simulink model "backupmodelforfutureuse24jan_2012b"  (R2012b)
settings: Solver=ode45  StartTime=0.0  StopTime=10.0  RelTol=1e-3
settings Model: Creator=Vicon  LastModifiedBy=Vicon

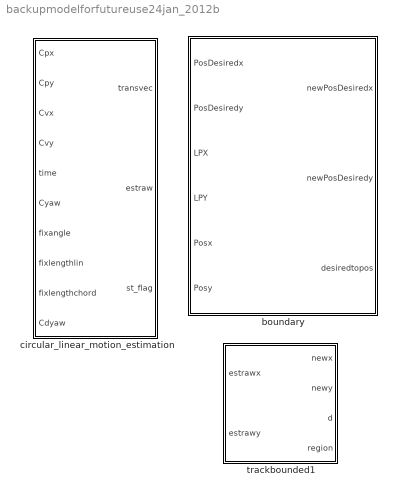
== system backupmodelforfutureuse24jan_2012b ==
  boundary : MATLAB Function  TreatAsAtomicUnit=on
  circular_linear_motion_estimation : MATLAB Function  TreatAsAtomicUnit=on
  trackbounded1 : MATLAB Function  TreatAsAtomicUnit=on

== matlab function backupmodelforfutureuse24jan_2012b/circular_linear_motion_estimation ==
  data: Cpx input; Cpy input; Cvx input; Cvy input; transvec output; estraw output; st_flag output; time input; Cyaw input; fixangle input; fixlengthlin input; fixlengthchord input; Cdyaw input
function [transvec,estraw,st_flag] = fcn(Cpx,Cpy,Cvx,Cvy,time,Cyaw,fixangle,fixlengthlin,fixlengthchord,Cdyaw)
if(Cvx == 0 && Cvy == 0)
    st_flag = 1;
else 
    st_flag = 0;
end
%%%%%%%%%%%%%%%%%%%%%%circular estimation%%%%%%%%%%%%%%%%%%%%%%%%%%%%
%vxyM = sqrt((Cvx)^2 + (Cvy)^2); %resultant vector vxy
if(st_flag == 0)
    
        angleOmega = Cyaw + 0.5 * fixangle * pi / 180; %angleOmega(radian): between vx and L
        zero_chk = 1;
else
    
      angleOmega = 0;  
      zero_chk = 0;
end
if(Cdyaw ~= 0) %use dyaw to select circular or linear estimation
%r = vxyM / abs(Cdyaw);
%Chord = 2 * r * sin(fixangle * pi / 360); %%%%%chord sometime will go to
%very large value, will disable this parameter soon
transveccir = [fixlengthchord * cos(angleOmega)*zero_chk  fixlengthchord * sin(angleOmega) * zero_chk];
transveclin = [0 0];
else
%%%%%%%%%%%%%%%%%%%%%%%%linear estimation%%%%%%%%%%%%%%%%%%%%%%%%%%%%%%
transveclin = [fixlengthlin * cos(Cyaw * pi / 180)*zero_chk fixlengthlin * sin(Cyaw * pi / 180)*zero_chk];
transveccir = [0 0];
%Chord = 0;
end
if(time<2)       %%%%%%%%%%%%%%%%%avoid noise when initializing the program in first 2 seconds
    transvec = [0 0];
else
transvec = transveccir + transveclin;
end

C2dvec = [Cpx Cpy];
estraw = C2dvec + transvec;

== matlab function backupmodelforfutureuse24jan_2012b/trackbounded1 ==
  data: newx output; newy output; estrawx input; estrawy input; d output; region output
function [newx,newy,d,region]  = fcn(estrawx,estrawy)
%#codegen
%cp = [cpy,cpx,0];
cpest = [estrawy, estrawx,0];
%%database of check points
chk0x = -0.4383;
chk0y = -0.9285;
chk1x = 1.047;
chk1y = -0.9693;
chk2x = 1.396;
chk2y = 0.4535;
chk3x = 1.382;
chk3y = 1.505;
chk4x = 1.042;
chk4y = 1.925;
chk5x = 0.3708;
chk5y = 1.821;
%%chk5x = ;
%%chk....
chk0 = [chk0y,chk0x,0];
chk1 = [chk1y,chk1x,0];
chk2 = [chk2y,chk2x,0];
chk3 = [chk3y,chk3x,0];
chk4 = [chk4y,chk4x,0];
chk5 = [chk5y,chk5x,0];
%%%%%%%%%%%%%%%%%%%%%%%%%%%%%%%%%%%%%%%%%%%%%%%%%%%%%%%%%%%%%%%%%%%%%%%%%%%%%%%%%%%%%%region selector
if(estrawx>2 && estrawx<=3 && estrawy>-3 && estrawy<=-2)
    region = 0;
elseif(estrawx>2 && estrawx<=3 && estrawy>-2 && estrawy<=-1 )
    region = 1;
elseif(estrawx>2 && estrawx<=3 && estrawy>-1 && estrawy<=0 )
    region = 2;
elseif(estrawx>2 && estrawx<=3 && estrawy>0 && estrawy<=1 )
    region = 3;
elseif(estrawx>2 && estrawx<=3 && estrawy>1 && estrawy<=2)
    region = 4;
elseif(estrawx>2 && estrawx<=3 && estrawy>2 && estrawy<=3)
    region = 5;
elseif(estrawx>1 && estrawx<=2 && estrawy>-3 && estrawy<=-2)
    region = 6;
elseif(estrawx>1 && estrawx<=2 && estrawy>-2 && estrawy<=-1)
    region = 7;
elseif(estrawx>1 && estrawx<=2 && estrawy>-1 && estrawy<=0)
    region = 8;
elseif(estrawx>1 && estrawx<=2 && estrawy>0 && estrawy<=1)
    region = 9;
elseif(estrawx>1 && estrawx<=2 && estrawy>1 && estrawy<=2)
    region = 10;
elseif(estrawx>1 && estrawx<=2 && estrawy>2 && estrawy<=3)
    region = 11;
elseif(estrawx>0 && estrawx<=1 && estrawy>-3 && estrawy<=-2)
    region = 12;
elseif(estrawx>0 && estrawx<=1 && estrawy>-2 && estrawy<=-1)
    region = 13;
elseif(estrawx>0 && estrawx<=1 && estrawy>-1 && estrawy<=0)
    region = 14;
elseif(estrawx>0 && estrawx<=1 && estrawy>0 && estrawy<=1)
    region = 15;
elseif(estrawx>0 && estrawx<=1 && estrawy>1 && estrawy<=2)
    region = 16;
elseif(estrawx>0 && estrawx<=1 && estrawy>2 && estrawy<=3)
    region = 17;
elseif(estrawx>-1 && estrawx<=0 && estrawy>-3 && estrawy<=-2)
    region = 18;
elseif(estrawx>-1 && estrawx<=0 && estrawy>-2 && estrawy<=-1)
    region = 19;
elseif(estrawx>-1 && estrawx<=0 && estrawy>-1 && estrawy<=0)
    region = 20;
elseif(estrawx>-1 && estrawx<=0 && estrawy>0 && estrawy<=1)
    region = 21;
elseif(estrawx>-1 && estrawx<=0 && estrawy>1 && estrawy<=2)
    region = 22;
elseif(estrawx>-1 && estrawx<=0 && estrawy>2 && estrawy<=3)
    region = 23;
elseif(estrawx>-2 && estrawx<=-1 && estrawy>-3 && estrawy<=-2)
    region = 24;
elseif(estrawx>-2 && estrawx<=-1 && estrawy>-2 && estrawy<=-1)
    region = 25;
elseif(estrawx>-2 && estrawx<=-1 && estrawy>-1 && estrawy<=0)
    region = 26;
elseif(estrawx>-2 && estrawx<=-1 && estrawy>0 && estrawy<=1)
    region = 27;
elseif(estrawx>-2 && estrawx<=-1 && estrawy>1 && estrawy<=2)
    region = 28;
elseif(estrawx>-2 && estrawx<=-1 && estrawy>2 && estrawy<=3)
    region = 29;
elseif(estrawx>-3 && estrawx<=-2 && estrawy>-3 && estrawy<=-2)
    region = 30;
elseif(estrawx>-3 && estrawx<=-2 && estrawy>-2 && estrawy<=-1)
    region = 31;
elseif(estrawx>-3 && estrawx<=-2 && estrawy>-1 && estrawy<=0)
    region = 32;
elseif(estrawx>-3 && estrawx<=-2 && estrawy>0 && estrawy<=1)
    region = 33;
elseif(estrawx>-3 && estrawx<=-2 && estrawy>1 && estrawy<=2)
    region = 34;
elseif(estrawx>-3 && estrawx<=-2 && estrawy>2 && estrawy<=3)
    region = 35;
else
    region = -1;
end
%%%%%%%%%%%%%%%%%%%%%%%%%%%%%%%%%%%%%%%%%%%%%%%%%%%%%%%%%%%%%%%%%%%%%%%%%%%%%%%%%%%%%%%%%%%%%%%%%%
if(region == 20 || region==19||region==13||region==14||region==7||region==21||region==6||region==12||region==18||region==24||region==25||region==26||region==27)
    %%%%%%%%%%%%%%%%calculate point to line distance%%%%%%%%%%%
    a = chk1 - chk0;
    b = cpest - chk0;
    d = norm(cross(a,b)) / norm(a);
    angle = atan2((chk1x-chk0x),(chk1y-chk0y));
    samplex = chk0x;
    sampley = chk0y;
    samplefinalx = chk1x;
    samplefinaly = chk1y;
    zero = 1;
elseif(region == 2||region==1||region==0||region==8)
    a = chk2 - chk1;
    b = cpest - chk1;
    d = norm(cross(a,b)) / norm(a);
    angle = atan2((chk2x-chk1x),(chk2y-chk1y));
    zero = 1;
    samplex = chk1x;
    sampley = chk1y;
    samplefinalx = chk2x;
    samplefinaly = chk2y;
elseif(region == 3||region==9||region==15)
    a = chk3 - chk2;
    b = cpest - chk2;
    d = norm(cross(a,b)) / norm(a);
    angle = atan2((chk3x-chk2x),(chk3y-chk2y));
    zero = 1;
    samplex = chk2x;
    sampley = chk2y;
    samplefinalx = chk3x;
    samplefinaly = chk3y;
elseif(region == 5||region==5||region==10||region==11)
    a = chk4 - chk3;
    b = cpest - chk3;
    d = norm(cross(a,b)) / norm(a);
    angle = atan2((chk4x-chk3x),(chk4y-chk3y));
    zero = 1;  
    samplex = chk3x;
    sampley = chk3y;
    samplefinalx = chk4x;
    samplefinaly = chk4y;
elseif(region == 16||region==17||region==22||region==23||region==28||region==29||region==34||region==35)
    a = chk5 - chk4;
    b = cpest - chk4;
    d = norm(cross(a,b)) / norm(a);
    angle = atan2((chk5x-chk4x),(chk5y-chk4y));
    zero = 1;
     samplex = chk4x;
    sampley = chk4y;
    samplefinalx = chk5x;
    samplefinaly = chk5y;

else
    a = -1;
    b = -1;
    d = -1;
    angle = -1;%%% i know this is not correct i will add one more zero coefficient to cancel this case
    zero = 0;
    samplex = 0;
    sampley = 0;
    samplefinalx = 0;
    samplefinaly = 0;
end
%%%%%%%%%%%%%%%%%%%%%%%%%%%%%%%%%%%%%%%%%%%%%%%%%%%%%%%%%%%%%%%%%%%%%%%%%%%%%%%%%%%%%%%%%%%%%%%%%%
%%calculate project point on the check point line
if(region == -1)%%if out of boundary none of the region match
        newy = 0;
        newx = 0;
else   %%match the region

distance = sqrt((samplefinalx-estrawx)^2+(samplefinaly-estrawy)^2); 
%if(distance > 1)
    %newx = samplefinalx;
   % newy = samplefinaly;
%else
      if(d<0.75)%%test the boundary width normal case if less than 0.75 m
    newx = estrawx;
    newy = estrawy;
      else%% out of boundary
        if(angle == 0 ||angle == 180)
            newx  = samplex;
            newy = estrawy;
        elseif(angle == 90 || angle == 270)
            newx = estrawx;
            newy = sampley;
        else
         kk = -1/(tan(angle));
         m = estrawx - kk*estrawy ;
         k = tan(angle);
         newy = (samplex - k*sampley - m)/(kk - k);
         newx = kk*newy + m;
        end
      end
%end
end

== matlab function backupmodelforfutureuse24jan_2012b/boundary ==
  data: PosDesiredx input; newPosDesiredx output; PosDesiredy input; LPX input; LPY input; Posx input; Posy input; newPosDesiredy output; desiredtopos output
function [newPosDesiredx, newPosDesiredy,desiredtopos] = fcn(PosDesiredx,PosDesiredy, LPX,LPY,Posx,Posy)

UAVreal = [Posy, Posx,0];
UAVdesired = [PosDesiredy, PosDesiredx,0];
LA = [LPY, LPX,0];
r = 1.2;%%%%%landing_area circle radius
%%%%%%%%%%%%%%%%calculate point to line distance%%%%%%%%%%%
if(PosDesiredx == Posx && PosDesiredy == Posy)
    d = 1.3; %%%%%%%%%%%whatever value larger than 1.2, just for if this is not a line but a point
else
    a = UAVdesired - UAVreal;
    b = LA - UAVreal;
    d = norm(cross(a,b)) / norm(a);
end
%%%%%%%%%%%%%%%%%%%%%%%%%%%%%%%%%%%%%%%%%%%%%%%%%%%%%%%%%%
k = (PosDesiredx-Posx)/(PosDesiredy-Posy);
m = -k*PosDesiredy + PosDesiredx - LPX;
desiredtopos = sqrt((PosDesiredy-Posy)^2+(PosDesiredx-Posx)^2);
w = 0;
angleLAtoPos=atan2((Posx-LPX),(Posy-LPY));
if((Posx-LPX)^2+(Posy-LPY)^2<=r^2)%%%uav inside the circle already
    newPosDesiredx = LPX + r*cos(angleLAtoPos);
    newPosDesiredy = LPY + r*sin(angleLAtoPos);
else%%%%%%%uav outside the circle
if(d>=r)%%outside or tangent with circle
    n = 0;
    w = 0;
    zerochk = 0;
    wperpendicular = (w + 0.5 * pi)*zerochk;
    intersecty1 = Posy;
    intersecty2 = Posy;
    intersectx1 = Posx;
    intersectx2 = Posx;
    intersec1topos = sqrt((intersecty1-Posy)^2 + (intersectx1-Posx)^2);
    intersec2topos = sqrt((intersecty2-Posy)^2 + (intersectx2-Posx)^2);
    newPosDesiredy = PosDesiredy;
    newPosDesiredx = PosDesiredx;
else 
    n = sqrt(4*(LPY - k*m)^2 - 4*(k^2+1)*(LPY^2 + m^2 - r^2));
    intersecty1 = (2*(LPY - k*m)+n)/(2*(k^2+1));
    intersecty2 = (2*(LPY - k*m)-n)/(2*(k^2+1));
    intersectx1 = k*(intersecty1 - PosDesiredy)+PosDesiredx;
    intersectx2 = k*(intersecty2 - PosDesiredy)+PosDesiredx;
    intersec1topos = sqrt((intersecty1-Posy)^2 + (intersectx1-Posx)^2);
    intersec2topos = sqrt((intersecty2-Posy)^2 + (intersectx2-Posx)^2);
    if(intersec1topos<intersec2topos)
        w = atan2((LPX-intersectx1),(LPY-intersecty1));
    else
        w = atan2((LPX-intersectx2),(LPY-intersecty2));
    end
        if(desiredtopos<=intersec1topos && desiredtopos<=intersec2topos)
            newPosDesiredx = PosDesiredx;
            newPosDesiredy = PosDesiredy;
            zerochk = 0;
            wperpendicular = (w + 0.5 * pi)*zerochk;
        elseif(desiredtopos<=intersec1topos && desiredtopos>intersec2topos)
            newPosDesiredx = intersectx2;
            newPosDesiredy = intersecty2;
            zerochk = 0;
            wperpendicular = (w + 0.5 * pi)*zerochk;
        elseif(desiredtopos>intersec1topos && desiredtopos<=intersec2topos)  
            newPosDesiredx = intersectx1;
            newPosDesiredy = intersecty1;
            zerochk = 0;
            wperpendicular = (w + 0.5 * pi)*zerochk;
        else
            zerochk = 1;
            wperpendicular = (w + 0.5 * pi)*zerochk;
            if(intersec1topos<intersec2topos)
            newPosDesiredx = 0.5*cos(wperpendicular) + intersectx1;
            newPosDesiredy = 0.5*sin(wperpendicular) + intersecty1;
            else
            newPosDesiredx = 0.5*cos(wperpendicular) + intersectx2;
            newPosDesiredy = 0.5*sin(wperpendicular) + intersecty2;  
            end
            
        end
    
end 
end
